simulink library "Plane_Movement_walk_forward"  (R2024a)
settings: Solver=VariableStepAuto  StartTime=0.0  StopTime=10.0  RelTol=1e-3
undefined symbols (not defined in the file): Lower_limbs, Upper_limbs
libraries: functionAngles x1, functionBezier_forward x1
settings Model: Creator=renre  LastModifiedBy=renre

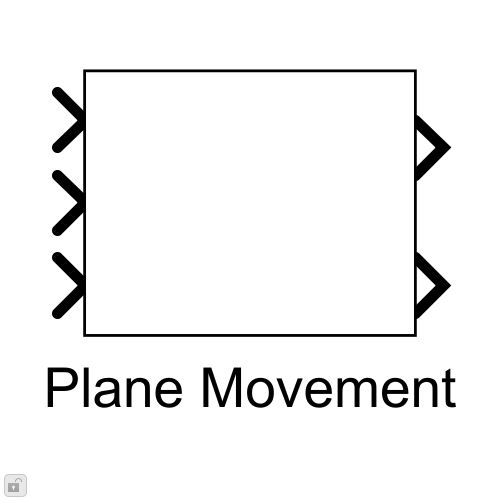
[thumbnail: Simulink's stored preview of the top-level diagram]
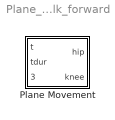
== system Plane_Movement_walk_forward ==
  Plane Movement : Subsystem

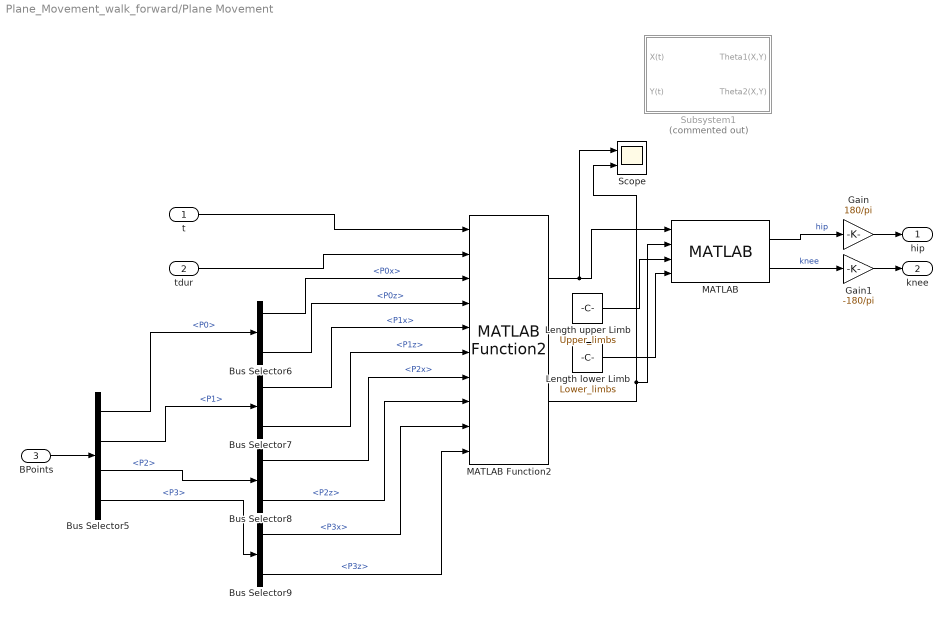
== system Plane_Movement_walk_forward/Plane Movement ==
  t : Inport
  tdur : Inport  Port=2
  BPoints : Inport  Port=3
  Bus Selector5 : BusSelector  OutputSignals=P0,P1,P2,P3
  Bus Selector6 : BusSelector  OutputSignals=P0x,P0y,P0z
  Bus Selector7 : BusSelector  OutputSignals=P1x,P1y,P1z
  Bus Selector8 : BusSelector  OutputSignals=P2x,P2y,P2z
  Bus Selector9 : BusSelector  OutputSignals=P3x,P3y,P3z
  Gain : Gain  Gain=180/pi
  Gain1 : Gain  Gain=-180/pi
  Length lower Limb : Constant  Value=Lower_limbs
  Length upper Limb : Constant  Value=Upper_limbs
  MATLAB : functionAngles/MATLAB  SystemSampleTime=-1  VariantActivationTime=update diagram  AllowFlexibleInterface=on  Latency=0  AutoFrameSizeCalculation=off
  MATLAB Function2 : functionBezier_forward/MATLAB Function2  SystemSampleTime=-1  VariantActivationTime=update diagram  AllowFlexibleInterface=on  Latency=0  AutoFrameSizeCalculation=off
  Scope : Scope  NumInputPorts=2
  Subsystem1 : Subsystem  Commented=on
  hip : Outport
  knee : Outport  Port=2
  wires:
  Bus Selector7/3 -> MATLAB Function2/6  "<P1z>"
  Bus Selector5/1 -> Bus Selector6/1  "<P0>"
  Bus Selector6/1 -> MATLAB Function2/3  "<P0x>"
  BPoints/1 -> Bus Selector5/1
  Bus Selector5/2 -> Bus Selector7/1  "<P1>"
  Bus Selector9/3 -> MATLAB Function2/10  "<P3z>"
  Bus Selector5/4 -> Bus Selector9/1  "<P3>"
  Bus Selector6/3 -> MATLAB Function2/4  "<P0z>"
  Bus Selector9/1 -> MATLAB Function2/9  "<P3x>"
  Bus Selector8/1 -> MATLAB Function2/7  "<P2x>"
  Bus Selector7/1 -> MATLAB Function2/5  "<P1x>"
  Bus Selector8/3 -> MATLAB Function2/8  "<P2z>"
  Bus Selector5/3 -> Bus Selector8/1  "<P2>"
  MATLAB Function2/2 -> MATLAB/2, Scope/2
  MATLAB Function2/1 -> MATLAB/1, Scope/1
  MATLAB/2 -> Gain1/1  "knee"
  tdur/1 -> MATLAB Function2/2
  MATLAB/1 -> Gain/1  "hip"
  t/1 -> MATLAB Function2/1
  Length upper Limb/1 -> MATLAB/3
  Length lower Limb/1 -> MATLAB/4
  Gain1/1 -> knee/1
  Gain/1 -> hip/1

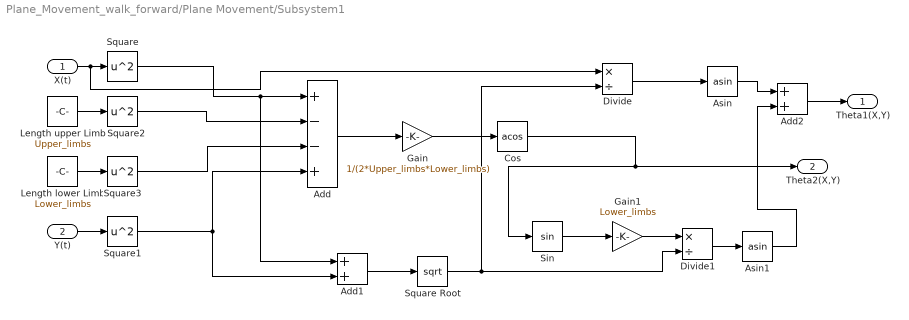
== system Plane_Movement_walk_forward/Plane Movement/Subsystem1 ==
  X(t) : Inport
  Y(t) : Inport  Port=2
  Add : Sum  Inputs=+--+
  Add1 : Sum
  Add2 : Sum
  Asin : Trigonometry  Operator=asin
  Asin1 : Trigonometry  Operator=asin
  Cos : Trigonometry  Operator=acos
  Divide : Product  Inputs=*/
  Divide1 : Product  Inputs=*/
  Gain : Gain  Gain=1/(2*Upper_limbs*Lower_limbs)
  Gain1 : Gain  Gain=Lower_limbs
  Length lower Limb : Constant  Value=Lower_limbs
  Length upper Limb : Constant  Value=Upper_limbs
  Sin : Trigonometry
  Square{,1..3} (4 alike) : Math  Operator=square
  Square Root : Sqrt
  Theta1(X,Y) : Outport
  Theta2(X,Y) : Outport  Port=2
  wires:
  X(t)/1 -> Divide/1, Square/1
  Y(t)/1 -> Square1/1
  Square/1 -> Add1/1, Add/1
  Length upper Limb/1 -> Square2/1
  Length lower Limb/1 -> Square3/1
  Square2/1 -> Add/2
  Square3/1 -> Add/3
  Square1/1 -> Add1/2, Add/4
  Add/1 -> Gain/1
  Gain/1 -> Cos/1
  Cos/1 -> Theta2(X,Y)/1, Sin/1
  Asin/1 -> Add2/1
  Sin/1 -> Gain1/1
  Add1/1 -> Square Root/1
  Gain1/1 -> Divide1/1
  Square Root/1 -> Divide/2, Divide1/2
  Divide1/1 -> Asin1/1
  Asin1/1 -> Add2/2
  Add2/1 -> Theta1(X,Y)/1
  Divide/1 -> Asin/1
